simulink model "BeispielBeobachter_1"  (Simulink 7.8)
settings: Solver=ode45  StartTime=0.0  StopTime=10  MaxStep=0.01  RelTol=1e-3
values from neighbouring files (symbols this model uses):
  a = 0    [Beobachterentwurf.m]
  h = TB*hB,    [Beobachterentwurf.m]
settings Model: Creator=Christoph Eck  LastModifiedBy=Chris
settings DataIOCC: SignalLoggingName=sigsOut
settings OptimizationCC: InitFltsAndDblsToZero=on
settings DebuggingCC: SaveWithParameterizedLinksMsg=none  SignalResolutionControl=TryResolveAllWithWarning  SolverPrmCheckMsg=none  MultiTaskDSMMsg=warning  MultiTaskCondExecSysMsg=none  FcnCallInpInsideContextMsg=Use local settings  StrictBusMsg=None
settings HardwareCC: TargetUnknown=on
settings RTWCC: IncludeERTFirstTime=on
settings GRTTargetCC: TargetFcnLib=ansi_tfl_tmw.mat

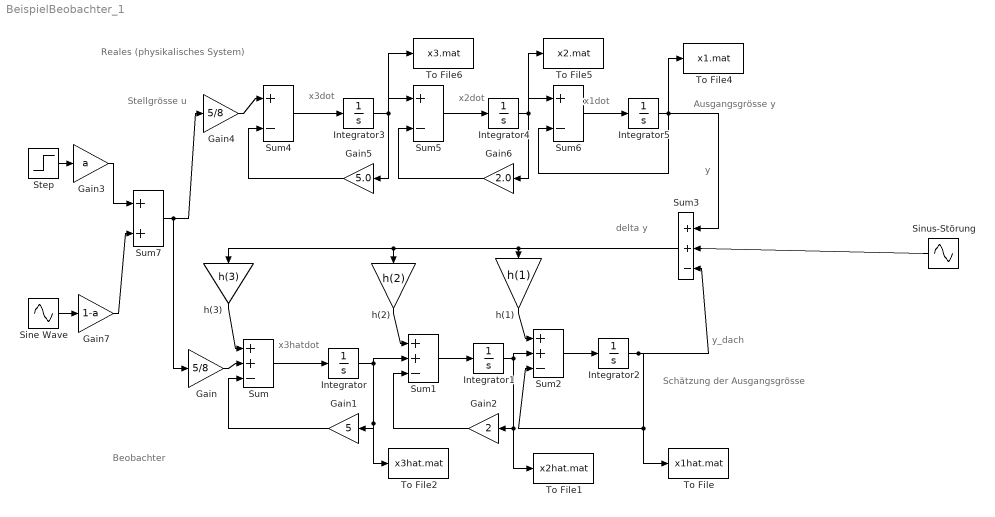
== system BeispielBeobachter_1 ==
  note: y_dach
  note: y
  note: x3dot
  note: x2dot
  note: x1dot
  note: Stellgrösse u
  note: Ausgangsgrösse y
  note: x3hatdot
  note: Schätzung der
      | Ausgangsgrösse
  note: delta y
  note: Reales (physikalisches System)
  note: Beobachter
  Gain : Gain  Gain=5/8  SaturateOnIntegerOverflow=on  OutDataTypeStr=Inherit: Same as input  ParamDataTypeStr=Inherit: Same as input
  Gain1 : Gain  Gain=5  SaturateOnIntegerOverflow=on  OutDataTypeStr=Inherit: Same as input  ParamDataTypeStr=Inherit: Same as input
  Gain2 : Gain  Gain=2  SaturateOnIntegerOverflow=on  OutDataTypeStr=Inherit: Same as input  ParamDataTypeStr=Inherit: Same as input
  Gain3 : Gain  Gain=a  SaturateOnIntegerOverflow=on  OutDataTypeStr=Inherit: Same as input  ParamDataTypeStr=Inherit: Same as input
  Gain4 : Gain  Gain=5/8  SaturateOnIntegerOverflow=on  OutDataTypeStr=Inherit: Same as input  ParamDataTypeStr=Inherit: Same as input
  Gain5 : Gain  Gain=5.0  SaturateOnIntegerOverflow=on  OutDataTypeStr=Inherit: Same as input  ParamDataTypeStr=Inherit: Same as input
  Gain6 : Gain  Gain=2.0  SaturateOnIntegerOverflow=on  OutDataTypeStr=Inherit: Same as input  ParamDataTypeStr=Inherit: Same as input
  Gain7 : Gain  Gain=1-a  SaturateOnIntegerOverflow=on  OutDataTypeStr=Inherit: Same as input  ParamDataTypeStr=Inherit: Same as input
  Integrator : Integrator  InitialCondition=5
  Integrator1 : Integrator  InitialCondition=-3
  Integrator2 : Integrator  InitialCondition=-10
  Integrator3 : Integrator  InitialCondition=1
  Integrator4 : Integrator  InitialCondition=1
  Integrator5 : Integrator  InitialCondition=2
  Sine Wave : Sin  Amplitude=2  SampleTime=0
  Sinus-Störung : Sin  Amplitude=0.1  Frequency=3  SampleTime=0
  Step : Step  Time=0  After=16  SampleTime=0
  Sum{,1..3} (4 alike) : Sum  Inputs=|++-  SaturateOnIntegerOverflow=on
  Sum4 : Sum  Inputs=|+-  SaturateOnIntegerOverflow=on
  Sum5 : Sum  Inputs=|+-  SaturateOnIntegerOverflow=on
  Sum6 : Sum  Inputs=|+-  SaturateOnIntegerOverflow=on
  Sum7 : Sum  SaturateOnIntegerOverflow=on
  To File : ToFile  Filename=x1hat.mat  MatrixName=x1hat
  To File1 : ToFile  Filename=x2hat.mat  MatrixName=x2hat
  To File2 : ToFile  Filename=x3hat.mat  MatrixName=x3hat
  To File4 : ToFile  Filename=x1.mat  MatrixName=x1
  To File5 : ToFile  Filename=x2.mat  MatrixName=x2
  To File6 : ToFile  Filename=x3.mat  MatrixName=x3
  h(1) : Gain  Gain=h(1)  SaturateOnIntegerOverflow=on  OutDataTypeStr=Inherit: Same as input  ParamDataTypeStr=Inherit: Same as input
  h(2) : Gain  Gain=h(2)  SaturateOnIntegerOverflow=on  OutDataTypeStr=Inherit: Same as input  ParamDataTypeStr=Inherit: Same as input
  h(3) : Gain  Gain=h(3)  SaturateOnIntegerOverflow=on  OutDataTypeStr=Inherit: Same as input  ParamDataTypeStr=Inherit: Same as input
  wires:
  Sum/1 -> Integrator/1
  Gain1/1 -> Sum/3
  Gain2/1 -> Sum1/3
  Gain/1 -> Sum/2
  Integrator/1 -> Sum1/2, To File2/1, Gain1/1
  Sum1/1 -> Integrator1/1
  Integrator1/1 -> Sum2/2, Gain2/1, To File1/1
  Sum2/1 -> Integrator2/1
  Integrator2/1 -> Sum2/3, To File/1, Sum3/3
  Sum4/1 -> Integrator3/1
  Gain5/1 -> Sum4/2
  Integrator3/1 -> Gain5/1, Sum5/1, To File6/1
  Sum5/1 -> Integrator4/1
  Integrator4/1 -> Gain6/1, Sum6/1, To File5/1
  Sum6/1 -> Integrator5/1
  Integrator5/1 -> Sum6/2, To File4/1, Sum3/1
  Sum3/1 -> h(3)/1, h(2)/1, h(1)/1
  h(3)/1 -> Sum/1
  h(2)/1 -> Sum1/1
  h(1)/1 -> Sum2/1
  Gain4/1 -> Sum4/1
  Gain6/1 -> Sum5/2
  Gain3/1 -> Sum7/1
  Step/1 -> Gain3/1
  Sine Wave/1 -> Gain7/1
  Sum7/1 -> Gain4/1, Gain/1
  Gain7/1 -> Sum7/2
  Sinus-Störung/1 -> Sum3/2
